simulink model "s2dot3_62"  (R2023b)
settings: Solver=VariableStepAuto  StartTime=0.0  StopTime=10.0  RelTol=1e-3
settings Model: Creator=lxj  LastModifiedBy=lxj

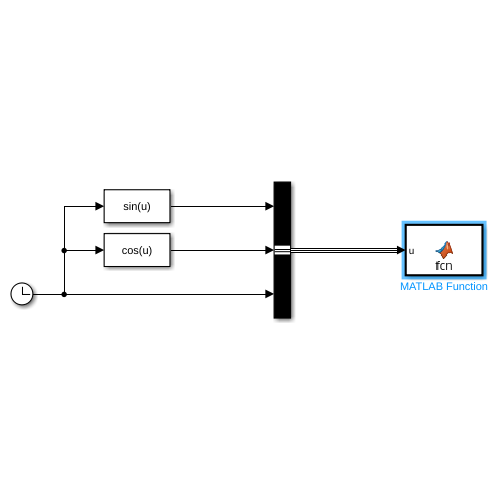
[thumbnail: Simulink's stored preview of the top-level diagram]
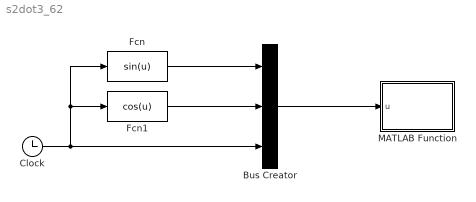
== system s2dot3_62 ==
  Bus Creator : BusCreator  Inputs=3
  Clock : Clock
  Fcn : Fcn  Expr=sin(u)
  Fcn1 : Fcn  Expr=cos(u)
  MATLAB Function : MATLAB Function  TreatAsAtomicUnit=on
  wires:
  Bus Creator/1 -> MATLAB Function/1(u)
  Fcn/1 -> Bus Creator/1
  Fcn1/1 -> Bus Creator/2
  Clock/1 -> Fcn/1, Fcn1/1, Bus Creator/3

== matlab function s2dot3_62/MATLAB Function ==
  data: u input
function fcn(u)
%#codegen
eml.extrinsic('plot3', 'scatter3', 'close', 'delete');
len = length(u);
persistent data;
if isempty(data)
    data = zeros(3,100000);
end
persistent n;
if isempty(n)
    n = 1;
else
    n = n + 1;
end
data(:,n) = u;
persistent h;
if isempty(h)
    h = plot3(data(1,:), data(2,:), data(3,:), 'o');
else
    delete(h);
    h = plot3(data(1,:), data(2,:), data(3,:), 'o');
end
